simulink model "Aula9_simulink"  (R2013b)
settings: Solver=ode45  StartTime=0.0  StopTime=10  MaxStep=0.05  RelTol=1e-3
values from neighbouring files (symbols this model uses):
  K_ctrl = K_lqr    [Aula9.m]
  Ke = Ke_2    [Aula9.m]
  ruido = 1    [Aula9.m]
  x_ini = [5 2.5 5 2.5]    [Aula9.m]
libraries: simulink x4
settings Model: Creator=ThiagoCordeiro  LastModifiedBy=ThiagoFelippe

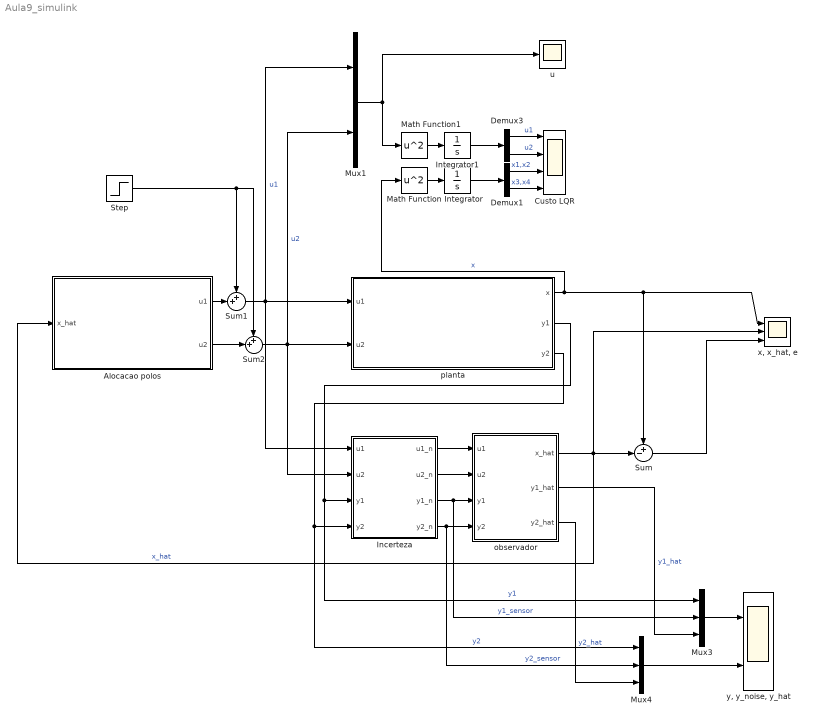
== system Aula9_simulink ==
  Alocacao polos : Subsystem
  Custo LQR : Scope  NumInputPorts=4
      settings: ShowLegends=on  YMin=-5~-5~-5~-5  YMax=5~5~5~5  SaveName=ScopeData5
  Demux1 : Demux  Outputs=2
  Demux3 : Demux  Outputs=2
  Incerteza : Subsystem
  Integrator : Integrator
  Integrator1 : Integrator
  Math Function : Math  Operator=square  SaturateOnIntegerOverflow=on
  Math Function1 : Math  Operator=square  SaturateOnIntegerOverflow=on
  Mux1 : Mux  Inputs=2
  Mux3 : Mux  Inputs=3
  Mux4 : Mux  Inputs=3
  Step : Step  After=0  SampleTime=0
  Sum : Sum  Inputs=+-|
  Sum1 : Sum  Inputs=++|
  Sum2 : Sum  Inputs=++|
  observador : Subsystem
  planta : Subsystem
  u : Scope
      settings: ShowLegends=on  TimeRange=10  SaveName=ScopeData3
  "x, x_hat, e" : Scope  NumInputPorts=3
      settings: ShowLegends=on  TimeRange=10  YMin=-80~-80~-5  YMax=60~40~5
  "y, y_noise, y_hat" : Scope  NumInputPorts=2
      settings: ShowLegends=on  YMin=-6.53629~-5  YMax=-6.47741~5
  wires:
  Math Function/1 -> Integrator/1
  Integrator/1 -> Demux1/1
  Demux1/1 -> Custo LQR/3  "x1,x2"
  Demux1/2 -> Custo LQR/4  "x3,x4"
  Mux1/1 -> Math Function1/1, u/1
  Math Function1/1 -> Integrator1/1
  Incerteza/1(u1_n) -> observador/1(u1)
  Incerteza/2(u2_n) -> observador/2(u2)
  Incerteza/3(y1_n) -> Mux3/2, observador/3(y1)  "y1_sensor"
  Incerteza/4(y2_n) -> Mux4/2, observador/4(y2)  "y2_sensor"
  planta/2(y1) -> Mux3/1, Incerteza/3(y1)  "y1"
  planta/3(y2) -> Mux4/1, Incerteza/4(y2)  "y2"
  observador/1(x_hat) -> "x, x_hat, e"/2, Sum/2, Alocacao polos/1(x_hat)  "x_hat"
  planta/1(x) -> Sum/1, "x, x_hat, e"/1, Math Function/1  "x"
  Demux3/1 -> Custo LQR/1  "u1"
  Demux3/2 -> Custo LQR/2  "u2"
  Integrator1/1 -> Demux3/1
  Mux3/1 -> "y, y_noise, y_hat"/1
  observador/2(y1_hat) -> Mux3/3  "y1_hat"
  Mux4/1 -> "y, y_noise, y_hat"/2
  observador/3(y2_hat) -> Mux4/3  "y2_hat"
  Alocacao polos/1(u1) -> Sum1/2
  Sum1/1 -> Incerteza/1(u1), planta/1(u1), Mux1/1  "u1"
  Alocacao polos/2(u2) -> Sum2/2
  Sum2/1 -> Incerteza/2(u2), planta/2(u2), Mux1/2  "u2"
  Step/1 -> Sum2/1, Sum1/1
  Sum/1 -> "x, x_hat, e"/3

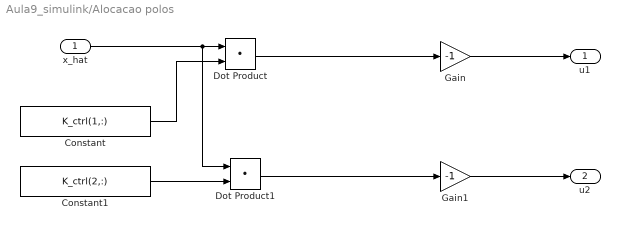
== system Aula9_simulink/Alocacao polos ==
  x_hat : Inport
  Constant : Constant  Value=K_ctrl(1,:)
  Constant1 : Constant  Value=K_ctrl(2,:)
  Dot Product : DotProduct  InputSameDT=on  OutDataTypeStr=Inherit: Inherit via internal rule
  Dot Product1 : DotProduct  InputSameDT=on  OutDataTypeStr=Inherit: Inherit via internal rule
  Gain : Gain  Gain=-1
  Gain1 : Gain  Gain=-1
  u1 : Outport
  u2 : Outport  Port=2
  wires:
  x_hat/1 -> Dot Product1/1, Dot Product/1
  Constant/1 -> Dot Product/2
  Constant1/1 -> Dot Product1/2
  Dot Product/1 -> Gain/1
  Gain/1 -> u1/1
  Dot Product1/1 -> Gain1/1
  Gain1/1 -> u2/1

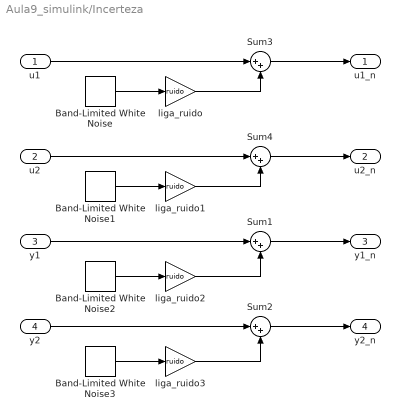
== system Aula9_simulink/Incerteza ==
  u1 : Inport
  u2 : Inport  Port=2
  y1 : Inport  Port=3
  y2 : Inport  Port=4
  Band-Limited White Noise : simulink/Sources/Band-Limited White Noise  Cov=[0.005]  Ts=0.01  seed=[23341]
  Band-Limited White Noise1 : simulink/Sources/Band-Limited White Noise  Cov=[0.005]  Ts=0.01  seed=[54321]
  Band-Limited White Noise2 : simulink/Sources/Band-Limited White Noise  Cov=[0.005]  Ts=0.01  seed=0
  Band-Limited White Noise3 : simulink/Sources/Band-Limited White Noise  Cov=[0.005]  Ts=0.01  seed=[14328]
  Sum{1..4} (4 alike) : Sum  Inputs=|++
  liga_ruido{,1..3} (4 alike) : Gain  Gain=ruido
  u1_n : Outport
  u2_n : Outport  Port=2
  y1_n : Outport  Port=3
  y2_n : Outport  Port=4
  wires:
  Sum1/1 -> y1_n/1
  Sum2/1 -> y2_n/1
  Sum4/1 -> u2_n/1
  Sum3/1 -> u1_n/1
  u1/1 -> Sum3/1
  u2/1 -> Sum4/1
  y1/1 -> Sum1/1
  y2/1 -> Sum2/1
  Band-Limited White Noise/1 -> liga_ruido/1
  liga_ruido/1 -> Sum3/2
  Band-Limited White Noise1/1 -> liga_ruido1/1
  liga_ruido1/1 -> Sum4/2
  Band-Limited White Noise2/1 -> liga_ruido2/1
  liga_ruido2/1 -> Sum1/2
  Band-Limited White Noise3/1 -> liga_ruido3/1
  liga_ruido3/1 -> Sum2/2

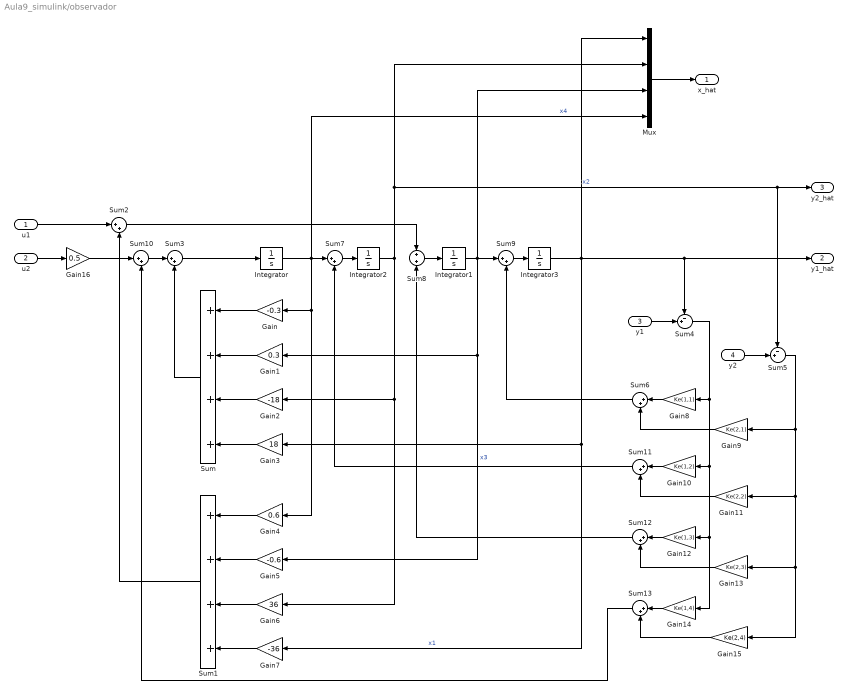
== system Aula9_simulink/observador ==
  u1 : Inport
  u2 : Inport  Port=2
  y1 : Inport  Port=3
  y2 : Inport  Port=4
  Gain : Gain  Gain=-0.3
  Gain1 : Gain  Gain=0.3
  Gain10 : Gain  Gain=Ke(1,2)
  Gain11 : Gain  Gain=Ke(2,2)
  Gain12 : Gain  Gain=Ke(1,3)
  Gain13 : Gain  Gain=Ke(2,3)
  Gain14 : Gain  Gain=Ke(1,4)
  Gain15 : Gain  Gain=Ke(2,4)
  Gain16 : Gain  Gain=0.5
  Gain2 : Gain  Gain=-18
  Gain3 : Gain  Gain=18
  Gain4 : Gain  Gain=0.6
  Gain5 : Gain  Gain=-0.6
  Gain6 : Gain  Gain=36
  Gain7 : Gain  Gain=-36
  Gain8 : Gain  Gain=Ke(1,1)
  Gain9 : Gain  Gain=Ke(2,1)
  Integrator{,1..3} (4 alike) : Integrator
  Mux : Mux
  Sum : Sum  Inputs=++++
  Sum1 : Sum  Inputs=++++
  Sum{2..3,6..7,9..13} (9 alike) : Sum  Inputs=|++
  Sum4 : Sum  Inputs=-+|
  Sum5 : Sum  Inputs=-+|
  Sum8 : Sum  Inputs=+|+
  x_hat : Outport
  y1_hat : Outport  Port=2
  y2_hat : Outport  Port=3
  wires:
  Gain/1 -> Sum/1
  Gain1/1 -> Sum/2
  Gain2/1 -> Sum/3
  Gain3/1 -> Sum/4
  Integrator/1 -> Sum7/1, Mux/4, Gain4/1, Gain/1  "x4"
  Integrator2/1 -> Gain6/1, Gain2/1, Mux/2, y2_hat/1, Sum5/1  "x2"
  Integrator3/1 -> y1_hat/1, Sum4/1, Gain7/1, Gain3/1, Mux/1  "x1"
  Gain4/1 -> Sum1/1
  Gain5/1 -> Sum1/2
  Gain6/1 -> Sum1/3
  Gain7/1 -> Sum1/4
  Integrator1/1 -> Sum9/1, Mux/3, Gain5/1, Gain1/1  "x3"
  Sum1/1 -> Sum2/2
  Sum3/1 -> Integrator/1
  Sum/1 -> Sum3/2
  u1/1 -> Sum2/1
  Mux/1 -> x_hat/1
  y1/1 -> Sum4/2
  y2/1 -> Sum5/2
  Sum5/1 -> Gain15/1, Gain13/1, Gain11/1, Gain9/1
  Gain8/1 -> Sum6/1
  Gain9/1 -> Sum6/2
  Sum7/1 -> Integrator2/1
  Sum2/1 -> Sum8/1
  Sum8/1 -> Integrator1/1
  Sum9/1 -> Integrator3/1
  Sum10/1 -> Sum3/1
  Sum6/1 -> Sum9/2
  Gain10/1 -> Sum11/1
  Gain11/1 -> Sum11/2
  Gain12/1 -> Sum12/1
  Gain13/1 -> Sum12/2
  Gain14/1 -> Sum13/1
  Gain15/1 -> Sum13/2
  Sum4/1 -> Gain14/1, Gain12/1, Gain10/1, Gain8/1
  Sum11/1 -> Sum7/2
  Sum12/1 -> Sum8/2
  Sum13/1 -> Sum10/2
  u2/1 -> Gain16/1
  Gain16/1 -> Sum10/1

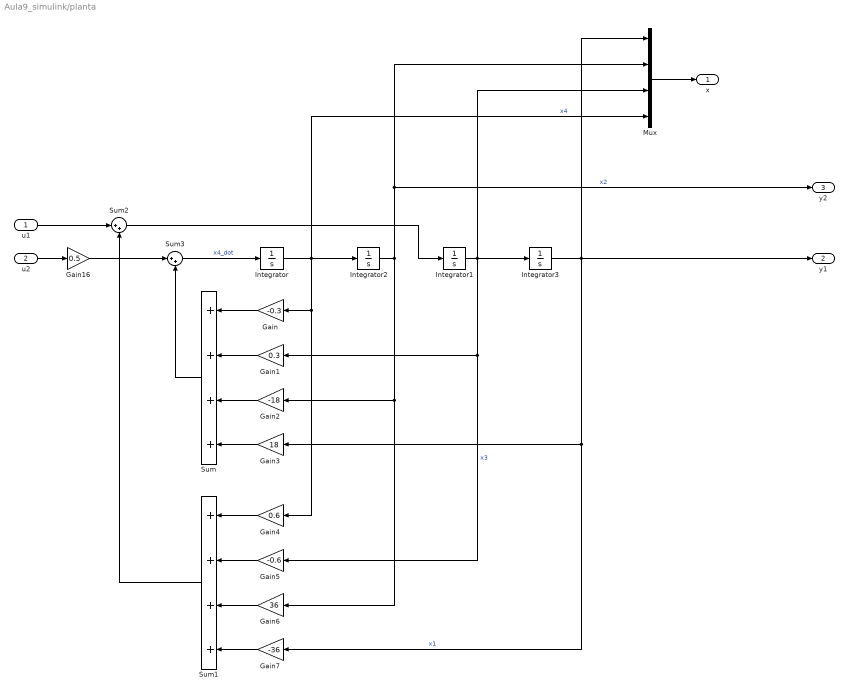
== system Aula9_simulink/planta ==
  u1 : Inport
  u2 : Inport  Port=2
  Gain : Gain  Gain=-0.3
  Gain1 : Gain  Gain=0.3
  Gain16 : Gain  Gain=0.5
  Gain2 : Gain  Gain=-18
  Gain3 : Gain  Gain=18
  Gain4 : Gain  Gain=0.6
  Gain5 : Gain  Gain=-0.6
  Gain6 : Gain  Gain=36
  Gain7 : Gain  Gain=-36
  Integrator : Integrator  InitialCondition=x_ini(4)
  Integrator1 : Integrator  InitialCondition=x_ini(3)
  Integrator2 : Integrator  InitialCondition=x_ini(2)
  Integrator3 : Integrator  InitialCondition=x_ini(1)
  Mux : Mux
  Sum : Sum  Inputs=++++
  Sum1 : Sum  Inputs=++++
  Sum2 : Sum  Inputs=|++
  Sum3 : Sum  Inputs=|++
  x : Outport
  y1 : Outport  Port=2
  y2 : Outport  Port=3
  wires:
  Gain/1 -> Sum/1
  Gain1/1 -> Sum/2
  Gain2/1 -> Sum/3
  Gain3/1 -> Sum/4
  Integrator/1 -> Integrator2/1, Mux/4, Gain4/1, Gain/1  "x4"
  Integrator2/1 -> Gain6/1, Gain2/1, Mux/2, y2/1  "x2"
  Integrator3/1 -> y1/1, Gain7/1, Gain3/1, Mux/1  "x1"
  Gain4/1 -> Sum1/1
  Gain5/1 -> Sum1/2
  Gain6/1 -> Sum1/3
  Gain7/1 -> Sum1/4
  Integrator1/1 -> Integrator3/1, Mux/3, Gain5/1, Gain1/1  "x3"
  Sum1/1 -> Sum2/2
  Sum3/1 -> Integrator/1  "x4_dot"
  Sum/1 -> Sum3/2
  u1/1 -> Sum2/1
  Mux/1 -> x/1
  Sum2/1 -> Integrator1/1
  Gain16/1 -> Sum3/1
  u2/1 -> Gain16/1
